simulink model "Main_Simulink"  (R2018b)
settings: Solver=VariableStepAuto  StartTime=0.0  StopTime=2.0  RelTol=1e-3  EnableMultiTasking=on
libraries: cstblocks x5, simulink_extras x1, RCTblocks x1
settings Model: Creator=duc  LastModifiedBy=auten
settings DataIOCC: LimitDataPoints=on
settings OptimizationCC: LifeSpan=inf
settings DebuggingCC: AllowSymbolicDim=off  SFUnexpectedBacktrackingDiag=warning  SFNoUnconditionalDefaultTransitionDiag=warning  SFExecutionAtInitializationDiag=none
settings ModelReferenceCC: PropagateSignalLabelsOutOfModel=off
settings SFSimCC: SimUseLocalCustomCode=off
settings RTWCC: RTWUseLocalCustomCode=off
settings CodeAppCC: StateflowObjectComments=on
settings GRTTargetCC: TargetLangStandard=C89/C90 (ANSI)
settings ConfigComp: CovMetricSettings=dw  CovHtmlReporting=on  CovSaveCumulativeToWorkspaceVar=on  CovSaveSingleToWorkspaceVar=on  CovExternalEMLEnable=off

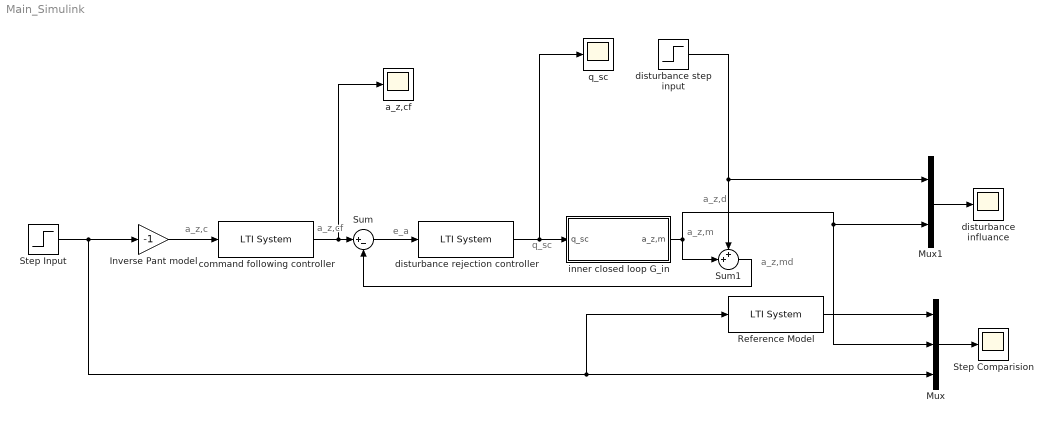
== system Main_Simulink ==
  note: a_z,c
  note: a_z,d
  note: a_z,md
  note: a_z,m
  note: q_sc
  note: e_a
  note: a_z,cf
  Inverse Pant model : Gain  Gain=-1
  Mux : Mux  Inputs=3
  Mux1 : Mux  Inputs=2
  Reference Model : cstblocks/LTI System  sys=T_r_m  IC=[]
  Step Comparision : Scope
  Step Input : Step  Time=0  SampleTime=0
  Sum : Sum  Inputs=|+-
  Sum1 : Sum  Inputs=++|
  a_z,cf : Scope
  command following controller : cstblocks/LTI System  sys=Kprime_cf  IC=[]
  disturbance influance : Scope
  disturbance rejection controller : cstblocks/LTI System  sys=Kprime_dr  IC=[]
  disturbance step input : Step  After=0.1  SampleTime=0
  "inner closed loop G_in " : Subsystem
  q_sc : Scope
  wires:
  disturbance rejection controller/1 -> "inner closed loop G_in "/1(q_sc), q_sc/1
  Sum/1 -> disturbance rejection controller/1
  "inner closed loop G_in "/1(a_z,m) -> Sum1/2, Mux/2, Mux1/2
  command following controller/1 -> Sum/1, a_z,cf/1
  Sum1/1 -> Sum/2
  Mux/1 -> Step Comparision/1
  Reference Model/1 -> Mux/1
  disturbance step input/1 -> Sum1/1, Mux1/1
  Step Input/1 -> Inverse Pant model/1, Reference Model/1, Mux/3
  Inverse Pant model/1 -> command following controller/1
  Mux1/1 -> disturbance influance/1

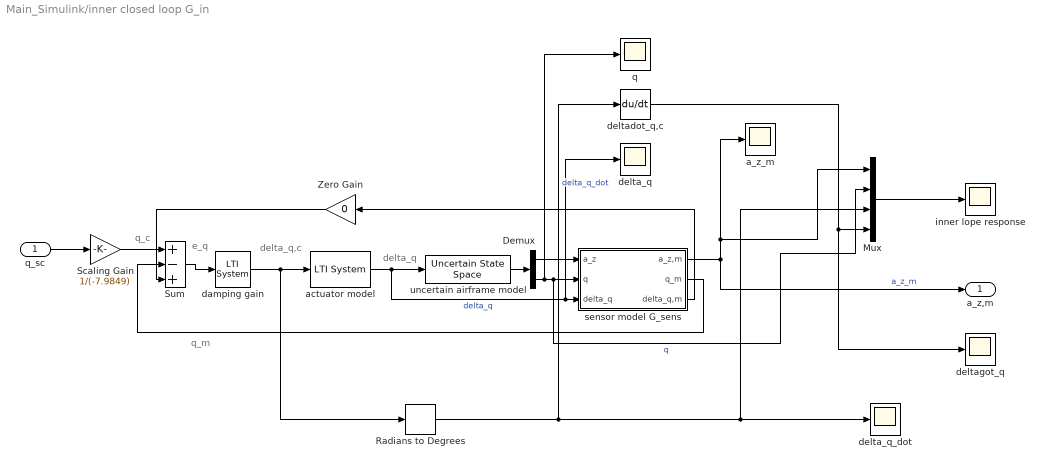
== system Main_Simulink/inner closed loop G_in  ==
  note: q_m
  note: q_c
  note: e_q
  note: delta_q,c
  note: delta_q
  q_sc : Inport
  Demux : Demux  Outputs=2
  Mux : Mux
  Radians to Degrees : simulink_extras/Transformations/Radians to Degrees
  Scaling Gain : Gain  Gain=1/(-7.9849)
  Sum : Sum  Inputs=+-+
  "Zero Gain " : Gain  Gain=0
  a_z_m : Scope
  actuator model : cstblocks/LTI System  sys=Gss_ac  IC=[]
  damping gain : cstblocks/LTI System  sys=K_q_sim  IC=[]
  delta_q : Scope
  "delta_q_dot " : Scope
  deltadot_q,c : Derivative
  deltagot_q : Scope
  inner lope response : Scope
  q : Scope
  sensor model G_sens : Subsystem
  uncertain airframe model : RCTblocks/Uncertain State Space  Tag=USS  USystem=Gss_af  UValue=Gss_af.Uncertainty  X0=[]  uX0=[]
      settings: SourceProductName=Robust Control Toolbox  SourceProductBaseCode=RC
  a_z,m : Outport
  wires:
  deltadot_q,c/1 -> deltagot_q/1, Mux/4
  Radians to Degrees/1 -> "delta_q_dot "/1, Mux/3, deltadot_q,c/1  "delta_q_dot"
  Demux/2 -> q/1, sensor model G_sens/2(q), Mux/2  "q"
  Mux/1 -> inner lope response/1
  "Zero Gain "/1 -> Sum/3
  sensor model G_sens/1(a_z,m) -> a_z,m/1, Mux/1, a_z_m/1  "a_z_m"
  q_sc/1 -> Scaling Gain/1
  sensor model G_sens/3(delta_q,m) -> "Zero Gain "/1
  sensor model G_sens/2(q_m) -> Sum/2
  Demux/1 -> sensor model G_sens/1(a_z)
  uncertain airframe model/1 -> Demux/1
  Sum/1 -> damping gain/1
  actuator model/1 -> uncertain airframe model/1, delta_q/1, sensor model G_sens/3(delta_q)  "delta_q"
  damping gain/1 -> Radians to Degrees/1, actuator model/1
  Scaling Gain/1 -> Sum/1

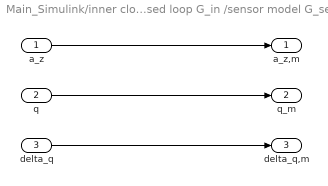
== system Main_Simulink/inner closed loop G_in /sensor model G_sens ==
  a_z : Inport
  q : Inport  Port=2
  delta_q : Inport  Port=3
  a_z,m : Outport
  q_m : Outport  Port=2
  delta_q,m : Outport  Port=3
  wires:
  delta_q/1 -> delta_q,m/1
  q/1 -> q_m/1
  a_z/1 -> a_z,m/1
